simulink model "master_thesis_simulink"  (R2022a)
settings: Solver=VariableStepAuto  StartTime=0.0  StopTime=p_0p.time(end)  FixedStep=0.001  RelTol=1e-3
values from neighbouring files (symbols this model uses):
  markers_forearm = [0.00210510253906 -0.143263397217 -0.00798474121094]    [markers_forearm.mat]
  markers_shoulder = [0.010127746582 -0.151647644043 -0.0119686279297]    [markers_shoulder.mat]
undefined symbols (not defined in the file or in its folder): arm, DiscIntNeverNeededParam, Discrete, ekf, kf, LS, m, markers_hand, n, noise, q0, q0_LS, q0_model, sample_Time, selected, state_observer, Time, tSh_0_0Conf, X, Y, Z
libraries: sm_lib x2029, nesl_utility x1553, robotlib x75, ctrlSharedLib x8
(part 32 of 70)

== system master_thesis_simulink/Experiments/S2_F0_H2/Model validation/Human arm/Wrist_joint ==
  note: Experiments
  Constant : Constant  Value=0
  Constant1 : Constant  Value=0
  Constant2 : Constant  Value=0
  F_elbow__Wx : Subsystem
  PS-Simulink Converter{1..3,9..11} (6 alike) : nesl_utility/PS-Simulink Converter  PhysicalDomain=network_engine_domain  SubClassName=ps_output  LeftPortType=input  RightPortType=output  PseudoPeriodic=off  Frequencies=[]  VectorFormat=inherit  Unit=inherit  AffineConversion=off
      settings: SourceProductBaseCode=SS,PW,VE
  RighForeArm_rot1 : sm_lib/Frames and Transforms/Rigid Transform  TranslationMethod=Cartesian  TranslationStandardOffset=0  TranslationLengthUnit=m  TranslationStandardAxis=+Z  TranslationCartesianOffset=[0 0 -arm.forearm.radius+arm.hand.dimensions(3)/2]  TranslationROffset=0  TranslationROffsetUnits=m  TranslationZOffset=0  TranslationZOffsetUnits=m  TranslationThetaOffset=0  TranslationThetaOffsetUnits=deg  RotationMethod=None  RotationAngleUnits=rad  RotationStandardAxis=+Z  RotationAngle=pi/2  RotationArbitraryAxis=[1 0 0]  FollAlignAxisA=+X  BaseAlignAxisA=+Y  FollAlignAxisB=+Y  BaseAlignAxisB=+Z  RotationSequenceAxes=BaseAxes  RotationSequence=XYZ  RotationSequenceAngles=[pi/2, 0, 0]  RotationSequenceAnglesUnits=rad  RotationMatrix=[1 0 0; 0 1 0; 0 0 1]
  Wx_Wy : Subsystem
  Wy_Wz : Subsystem
  c1 : nesl_utility/Simulink-PS Converter  PhysicalDomain=network_engine_domain  SubClassName=ps_input  LeftPortType=input  RightPortType=output  PseudoPeriodic=off  Frequencies=[]  NoiseDistribution=none  NoiseParameters=[]  Unit=1  AffineConversion=off  FilteringAndDerivatives=filter  SimscapeFilterOrder=2  InputFilterTimeConstant=0.001  UdotUserProvided=0
      settings: SourceProductBaseCode=SS,PW,VE
  c2 : nesl_utility/Simulink-PS Converter  PhysicalDomain=network_engine_domain  SubClassName=ps_input  LeftPortType=input  RightPortType=output  PseudoPeriodic=off  Frequencies=[]  NoiseDistribution=none  NoiseParameters=[]  Unit=1  AffineConversion=off  FilteringAndDerivatives=filter  SimscapeFilterOrder=2  InputFilterTimeConstant=0.001  UdotUserProvided=0
      settings: SourceProductBaseCode=SS,PW,VE
  c3 : nesl_utility/Simulink-PS Converter  PhysicalDomain=network_engine_domain  SubClassName=ps_input  LeftPortType=input  RightPortType=output  PseudoPeriodic=off  Frequencies=[]  NoiseDistribution=none  NoiseParameters=[]  Unit=1  AffineConversion=off  FilteringAndDerivatives=filter  SimscapeFilterOrder=2  InputFilterTimeConstant=0.001  UdotUserProvided=0
      settings: SourceProductBaseCode=SS,PW,VE
  jRightWrist_rotx : sm_lib/Joints/Revolute Joint  JointMode=Normal  SenseConstraintForce=off  SenseConstraintForceX=off  SenseConstraintForceY=off  SenseConstraintForceZ=off  SenseConstraintTorque=off  SenseConstraintTorqueX=off  SenseConstraintTorqueY=off  SenseConstraintTorqueZ=off  SenseTotalForce=off  SenseTotalForceX=off  SenseTotalForceY=off  SenseTotalForceZ=off  SenseTotalTorque=off  SenseTotalTorqueX=off  SenseTotalTorqueY=off  SenseTotalTorqueZ=off  CompositeWrenchDir=FollowerOnBase  CompositeWrenchFrame=BaseFrame  EquilibriumPosition=0  EquilibriumPositionUnits=deg  SpringStiffness=0  SpringStiffnessUnits=N*m/deg  DampingCoefficient=0.01  DampingCoefficientUnits=kg*m^2/(rad*s)  TorqueActuationMode=ComputedTorque  MotionActuationMode=InputMotion  SensePosition=on  SenseVelocity=on  SenseAcceleration=off  SenseTorqueForce=off  SenseLowerLimitTorqueForce=off  SenseUpperLimitTorqueForce=off  LowerLimitSpecify=on  LowerLimitBound=-pi/4  LowerLimitBoundUnits=rad  LowerLimitStiffness=1e4  LowerLimitStiffnessUnits=N*m/deg  LowerLimitDamping=10  LowerLimitDampingUnits=N*m/(deg/s)  LowerLimitTransitionRegionWidth=0.1  LowerLimitTransitionRegionWidthUnits=deg  UpperLimitSpecify=on  UpperLimitBound=pi/3  UpperLimitBoundUnits=rad  UpperLimitStiffness=1e4  UpperLimitStiffnessUnits=N*m/deg  UpperLimitDamping=10  UpperLimitDampingUnits=N*m/(deg/s)  UpperLimitTransitionRegionWidth=0.1  UpperLimitTransitionRegionWidthUnits=deg  PositionTargetSpecify=on  PositionTargetPriority=High  PositionTargetValue=0  PositionTargetValueUnits=rad  VelocityTargetSpecify=off  VelocityTargetPriority=High  VelocityTargetValue=0  VelocityTargetValueUnits=deg/s
  jRightWrist_roty : sm_lib/Joints/Revolute Joint  JointMode=Normal  SenseConstraintForce=off  SenseConstraintForceX=off  SenseConstraintForceY=off  SenseConstraintForceZ=off  SenseConstraintTorque=off  SenseConstraintTorqueX=off  SenseConstraintTorqueY=off  SenseConstraintTorqueZ=off  SenseTotalForce=off  SenseTotalForceX=off  SenseTotalForceY=off  SenseTotalForceZ=off  SenseTotalTorque=off  SenseTotalTorqueX=off  SenseTotalTorqueY=off  SenseTotalTorqueZ=off  CompositeWrenchDir=FollowerOnBase  CompositeWrenchFrame=BaseFrame  EquilibriumPosition=0  EquilibriumPositionUnits=deg  SpringStiffness=0  SpringStiffnessUnits=N*m/deg  DampingCoefficient=0  DampingCoefficientUnits=kg*m^2/(rad*s)  TorqueActuationMode=ComputedTorque  MotionActuationMode=InputMotion  SensePosition=on  SenseVelocity=on  SenseAcceleration=off  SenseTorqueForce=off  SenseLowerLimitTorqueForce=off  SenseUpperLimitTorqueForce=off  LowerLimitSpecify=on  LowerLimitBound=-pi/10  LowerLimitBoundUnits=rad  LowerLimitStiffness=1e4  LowerLimitStiffnessUnits=N*m/deg  LowerLimitDamping=10  LowerLimitDampingUnits=N*m/(deg/s)  LowerLimitTransitionRegionWidth=0.1  LowerLimitTransitionRegionWidthUnits=deg  UpperLimitSpecify=on  UpperLimitBound=pi/10  UpperLimitBoundUnits=rad  UpperLimitStiffness=1e4  UpperLimitStiffnessUnits=N*m/deg  UpperLimitDamping=10  UpperLimitDampingUnits=N*m/(deg/s)  UpperLimitTransitionRegionWidth=0.1  UpperLimitTransitionRegionWidthUnits=deg  PositionTargetSpecify=on  PositionTargetPriority=High  PositionTargetValue=0  PositionTargetValueUnits=rad  VelocityTargetSpecify=off  VelocityTargetPriority=High  VelocityTargetValue=0  VelocityTargetValueUnits=deg/s
  jRightWrist_rotz : sm_lib/Joints/Revolute Joint  JointMode=Normal  SenseConstraintForce=off  SenseConstraintForceX=off  SenseConstraintForceY=off  SenseConstraintForceZ=off  SenseConstraintTorque=off  SenseConstraintTorqueX=off  SenseConstraintTorqueY=off  SenseConstraintTorqueZ=off  SenseTotalForce=off  SenseTotalForceX=off  SenseTotalForceY=off  SenseTotalForceZ=off  SenseTotalTorque=off  SenseTotalTorqueX=off  SenseTotalTorqueY=off  SenseTotalTorqueZ=off  CompositeWrenchDir=FollowerOnBase  CompositeWrenchFrame=BaseFrame  EquilibriumPosition=0  EquilibriumPositionUnits=deg  SpringStiffness=0  SpringStiffnessUnits=N*m/deg  DampingCoefficient=0  DampingCoefficientUnits=kg*m^2/(rad*s)  TorqueActuationMode=ComputedTorque  MotionActuationMode=InputMotion  SensePosition=on  SenseVelocity=on  SenseAcceleration=off  SenseTorqueForce=off  SenseLowerLimitTorqueForce=off  SenseUpperLimitTorqueForce=off  LowerLimitSpecify=on  LowerLimitBound=-20  LowerLimitBoundUnits=deg  LowerLimitStiffness=1e4  LowerLimitStiffnessUnits=N*m/deg  LowerLimitDamping=10  LowerLimitDampingUnits=N*m/(deg/s)  LowerLimitTransitionRegionWidth=0.1  LowerLimitTransitionRegionWidthUnits=deg  UpperLimitSpecify=on  UpperLimitBound=pi/6  UpperLimitBoundUnits=rad  UpperLimitStiffness=1e4  UpperLimitStiffnessUnits=N*m/deg  UpperLimitDamping=10  UpperLimitDampingUnits=N*m/(deg/s)  UpperLimitTransitionRegionWidth=0.1  UpperLimitTransitionRegionWidthUnits=deg  PositionTargetSpecify=on  PositionTargetPriority=High  PositionTargetValue=0  PositionTargetValueUnits=rad  VelocityTargetSpecify=off  VelocityTargetPriority=High  VelocityTargetValue=0  VelocityTargetValueUnits=deg/s
  B_wrist : PMIOPort  Side=Right
  F_elbow : PMIOPort  Port=2  Side=Left
  tag scope: q5=global, q6=global, q7=global, qdot5=global, qdot6=global, qdot7=global
  wires:
  Constant2/1 -> c3/1
  Constant1/1 -> c2/1
  Constant/1 -> c1/1
  PS-Simulink Converter3/1 -> [qdot7]
  PS-Simulink Converter2/1 -> [qdot6]
  PS-Simulink Converter1/1 -> [qdot5]
  PS-Simulink Converter9/1 -> [q5]
  PS-Simulink Converter10/1 -> [q6]
  PS-Simulink Converter11/1 -> [q7]
  connections:
  RighForeArm_rot1/LConn1 -- F_elbow/RConn1
  c3/RConn1 -- jRightWrist_rotz/LConn2
  c2/RConn1 -- jRightWrist_roty/LConn2
  c1/RConn1 -- jRightWrist_rotx/LConn2
  ?
  ?
  ?
  jRightWrist_rotz/RConn3 -- PS-Simulink Converter3/LConn1
  jRightWrist_roty/RConn3 -- PS-Simulink Converter2/LConn1
  jRightWrist_rotx/RConn3 -- PS-Simulink Converter1/LConn1
  B_wrist/RConn1 -- jRightWrist_rotz/RConn1
  F_elbow__Wx/LConn1 -- RighForeArm_rot1/RConn1
  jRightWrist_roty/RConn1 -- Wy_Wz/LConn1
  PS-Simulink Converter9/LConn1 -- jRightWrist_rotx/RConn2
  PS-Simulink Converter10/LConn1 -- jRightWrist_roty/RConn2
  jRightWrist_roty/LConn1 -- Wx_Wy/RConn1
  jRightWrist_rotz/RConn2 -- PS-Simulink Converter11/LConn1
  Wy_Wz/RConn1 -- jRightWrist_rotz/LConn1
  jRightWrist_rotx/RConn1 -- Wx_Wy/LConn1
  F_elbow__Wx/RConn1 -- jRightWrist_rotx/LConn1

== system master_thesis_simulink/Ros2Matlab/S0_F1_H2/Subscriber/M0/Odom ==
  Bus Selector : BusSelector  OutputSignals=Pose.Covariance
  Bus Selector1 : BusSelector  OutputSignals=Twist.Covariance
  Bus1 : BusSelector  OutputSignals=Twist.Twist.Linear.X,Twist.Twist.Linear.Y,Twist.Twist.Linear.Z
  Mux2 : Mux  Inputs=3
  Subscribe_odom : robotlib/Subscribe  topicSource=Select from ROS network  topic=/qualisys/Super_marker_0/odom  messageType=nav_msgs/Odometry  SampleTime=sample_Time  legacyBusStruct=off  messageQueueLength=1
  Terminator3 : Terminator
  v0_W : Outport
  Rp0_W : Outport  Port=2
  Rv0_W : Outport  Port=3
  wires:
  Bus1/3 -> Mux2/3  "<Z>"
  Bus1/1 -> Mux2/1  "<X>"
  Bus1/2 -> Mux2/2  "<Y>"
  Subscribe_odom/1 -> Terminator3/1
  Mux2/1 -> v0_W/1
  Subscribe_odom/2 -> Bus Selector1/1, Bus Selector/1, Bus1/1
  Bus Selector/1 -> Rp0_W/1  "<Covariance>"
  Bus Selector1/1 -> Rv0_W/1  "<Covariance>"

== system master_thesis_simulink/Ros2Matlab/S0_F1_H2/Subscriber/M0/Pose ==
  Bus Selector : BusSelector  OutputSignals=Pose.Orientation.W
  Bus Selector1 : BusSelector  OutputSignals=Pose.Orientation.X
  Bus Selector2 : BusSelector  OutputSignals=Pose.Orientation.Y
  Bus Selector3 : BusSelector  OutputSignals=Pose.Position.X,Pose.Position.Y,Pose.Position.Z
  Bus Selector4 : BusSelector  OutputSignals=Pose.Orientation.Z
  Mux1 : Mux  Inputs=3
  Mux2 : Mux
  Subscribe_pose : robotlib/Subscribe  topicSource=Select from ROS network  topic=/qualisys/Super_marker_0/pose  messageType=geometry_msgs/PoseStamped  SampleTime=sample_Time  legacyBusStruct=off  messageQueueLength=1
  quat_02W : Outport
  p0_W : Outport  Port=2
  tag scope: M0_isNew=global
  wires:
  Mux2/1 -> quat_02W/1
  Bus Selector4/1 -> Mux2/4  "<Z>"
  Mux1/1 -> p0_W/1
  Bus Selector3/3 -> Mux1/3  "<Z>"
  Bus Selector3/2 -> Mux1/2  "<Y>"
  Bus Selector3/1 -> Mux1/1  "<X>"
  Bus Selector2/1 -> Mux2/3  "<Y>"
  Bus Selector1/1 -> Mux2/2  "<X>"
  Bus Selector/1 -> Mux2/1  "<W>"
  Subscribe_pose/2 -> Bus Selector/1, Bus Selector1/1, Bus Selector2/1, Bus Selector3/1, Bus Selector4/1
  Subscribe_pose/1 -> [M0_isNew]

== system master_thesis_simulink/Ros2Matlab/S0_F1_H2/Subscriber/M2/Odom ==
  Bus1 : BusSelector  OutputSignals=Twist.Twist.Linear.X,Twist.Twist.Linear.Y,Twist.Twist.Linear.Z
  Bus2 : BusSelector  OutputSignals=Pose.Covariance
  Bus3 : BusSelector  OutputSignals=Twist.Covariance
  Mux2 : Mux  Inputs=3
  Subscribe_twist : robotlib/Subscribe  topicSource=Select from ROS network  topic=/qualisys/Super_marker_2/odom  messageType=nav_msgs/Odometry  SampleTime=sample_Time  legacyBusStruct=off  messageQueueLength=1
  Terminator3 : Terminator
  v2_W : Outport
  Rp2_W : Outport  Port=2
  Rv2_W : Outport  Port=3
  wires:
  Mux2/1 -> v2_W/1
  Subscribe_twist/1 -> Terminator3/1
  Bus1/2 -> Mux2/2  "<Y>"
  Bus1/1 -> Mux2/1  "<X>"
  Bus1/3 -> Mux2/3  "<Z>"
  Bus2/1 -> Rp2_W/1  "<Covariance>"
  Subscribe_twist/2 -> Bus3/1, Bus2/1, Bus1/1
  Bus3/1 -> Rv2_W/1  "<Covariance>"

== system master_thesis_simulink/Ros2Matlab/S0_F1_H2/Subscriber/M2/Pose ==
  Bus : BusSelector  OutputSignals=Pose.Position.X,Pose.Position.Y,Pose.Position.Z
  Mux : Mux  Inputs=3
  Subscribe_pose : robotlib/Subscribe  topicSource=Select from ROS network  topic=/qualisys/Super_marker_2/pose  messageType=geometry_msgs/PoseStamped  SampleTime=sample_Time  legacyBusStruct=off  messageQueueLength=1
  p2_W : Outport
  tag scope: M2_isNew=global
  wires:
  Bus/2 -> Mux/2  "<Y>"
  Bus/3 -> Mux/3  "<Z>"
  Subscribe_pose/2 -> Bus/1
  Mux/1 -> p2_W/1
  Bus/1 -> Mux/1  "<X>"
  Subscribe_pose/1 -> [M2_isNew]

== system master_thesis_simulink/Ros2Matlab/S0_F1_H2/Subscriber/M3/Odom ==
  Bus1 : BusSelector  OutputSignals=Twist.Twist.Linear.X,Twist.Twist.Linear.Y,Twist.Twist.Linear.Z
  Bus2 : BusSelector  OutputSignals=Pose.Covariance
  Bus3 : BusSelector  OutputSignals=Twist.Covariance
  Mux2 : Mux  Inputs=3
  Subscribe_twist : robotlib/Subscribe  topicSource=Select from ROS network  topic=/qualisys/Super_marker_3/odom  messageType=nav_msgs/Odometry  SampleTime=sample_Time  legacyBusStruct=off  messageQueueLength=1
  Terminator3 : Terminator
  v3_W : Outport
  Rp3_W : Outport  Port=2
  Rv3_W : Outport  Port=3
  wires:
  Bus1/3 -> Mux2/3  "<Z>"
  Bus1/1 -> Mux2/1  "<X>"
  Bus1/2 -> Mux2/2  "<Y>"
  Subscribe_twist/1 -> Terminator3/1
  Mux2/1 -> v3_W/1
  Bus2/1 -> Rp3_W/1  "<Covariance>"
  Subscribe_twist/2 -> Bus3/1, Bus2/1, Bus1/1
  Bus3/1 -> Rv3_W/1  "<Covariance>"

== system master_thesis_simulink/Ros2Matlab/S0_F1_H2/Subscriber/M3/Pose ==
  Bus : BusSelector  OutputSignals=Pose.Position.X,Pose.Position.Y,Pose.Position.Z
  Mux : Mux  Inputs=3
  Subscribe_pose : robotlib/Subscribe  topicSource=Select from ROS network  topic=/qualisys/Super_marker_3/pose  messageType=geometry_msgs/PoseStamped  SampleTime=sample_Time  legacyBusStruct=off  messageQueueLength=1
  p3_W : Outport
  tag scope: M3_isNew=global
  wires:
  Bus/1 -> Mux/1  "<X>"
  Mux/1 -> p3_W/1
  Subscribe_pose/2 -> Bus/1
  Bus/3 -> Mux/3  "<Z>"
  Bus/2 -> Mux/2  "<Y>"
  Subscribe_pose/1 -> [M3_isNew]

== system master_thesis_simulink/Ros2Matlab/S0_F1_H2/Subscriber/M4/Odom ==
  Bus1 : BusSelector  OutputSignals=Twist.Twist.Linear.X,Twist.Twist.Linear.Y,Twist.Twist.Linear.Z
  Bus2 : BusSelector  OutputSignals=Pose.Covariance
  Bus3 : BusSelector  OutputSignals=Twist.Covariance
  Mux2 : Mux  Inputs=3
  Subscribe_twist : robotlib/Subscribe  topicSource=Select from ROS network  topic=/qualisys/Super_marker_4/odom  messageType=nav_msgs/Odometry  SampleTime=sample_Time  legacyBusStruct=off  messageQueueLength=1
  Terminator3 : Terminator
  v4_W : Outport
  Rp4_W : Outport  Port=2
  Rv4_W : Outport  Port=3
  wires:
  Mux2/1 -> v4_W/1
  Subscribe_twist/1 -> Terminator3/1
  Bus1/2 -> Mux2/2  "<Y>"
  Bus1/1 -> Mux2/1  "<X>"
  Bus1/3 -> Mux2/3  "<Z>"
  Subscribe_twist/2 -> Bus3/1, Bus2/1, Bus1/1
  Bus2/1 -> Rp4_W/1  "<Covariance>"
  Bus3/1 -> Rv4_W/1  "<Covariance>"

== system master_thesis_simulink/Ros2Matlab/S0_F1_H2/Subscriber/M4/Pose ==
  Bus : BusSelector  OutputSignals=Pose.Position.X,Pose.Position.Y,Pose.Position.Z
  Mux : Mux  Inputs=3
  Subscribe_pose : robotlib/Subscribe  topicSource=Select from ROS network  topic=/qualisys/Super_marker_4/pose  messageType=geometry_msgs/PoseStamped  SampleTime=sample_Time  legacyBusStruct=off  messageQueueLength=1
  p4_W : Outport
  tag scope: M4_isNew=global
  wires:
  Bus/2 -> Mux/2  "<Y>"
  Bus/3 -> Mux/3  "<Z>"
  Subscribe_pose/2 -> Bus/1
  Mux/1 -> p4_W/1
  Bus/1 -> Mux/1  "<X>"
  Subscribe_pose/1 -> [M4_isNew]

== system master_thesis_simulink/Ros2Matlab/S0_F1_H2/Subscriber/Shoulder_RF/Pose ==
  Bus Selector : BusSelector  OutputSignals=Pose.Orientation.W
  Bus Selector1 : BusSelector  OutputSignals=Pose.Orientation.X
  Bus Selector2 : BusSelector  OutputSignals=Pose.Orientation.Y
  Bus Selector3 : BusSelector  OutputSignals=Pose.Position.X,Pose.Position.Y,Pose.Position.Z
  Bus Selector4 : BusSelector  OutputSignals=Pose.Orientation.Z
  Mux1 : Mux  Inputs=3
  Mux2 : Mux
  Subscribe_pose : robotlib/Subscribe  topicSource=Select from ROS network  topic=/qualisys/Shoulder_RF/pose  messageType=geometry_msgs/PoseStamped  SampleTime=sample_Time  legacyBusStruct=off  messageQueueLength=1
  quat_Sh2W : Outport
  pSh_W : Outport  Port=2
  tag scope: Sh_isNew=global
  wires:
  Mux2/1 -> quat_Sh2W/1
  Bus Selector4/1 -> Mux2/4  "<Z>"
  Mux1/1 -> pSh_W/1
  Bus Selector3/3 -> Mux1/3  "<Z>"
  Bus Selector3/2 -> Mux1/2  "<Y>"
  Bus Selector3/1 -> Mux1/1  "<X>"
  Bus Selector2/1 -> Mux2/3  "<Y>"
  Bus Selector1/1 -> Mux2/2  "<X>"
  Bus Selector/1 -> Mux2/1  "<W>"
  Subscribe_pose/2 -> Bus Selector/1, Bus Selector1/1, Bus Selector2/1, Bus Selector3/1, Bus Selector4/1
  Subscribe_pose/1 -> [Sh_isNew]

== system master_thesis_simulink/Ros2Matlab/S0_F2_H2/Subscriber/M0/Odom ==
  Bus Selector : BusSelector  OutputSignals=Pose.Covariance
  Bus Selector1 : BusSelector  OutputSignals=Twist.Covariance
  Bus1 : BusSelector  OutputSignals=Twist.Twist.Linear.X,Twist.Twist.Linear.Y,Twist.Twist.Linear.Z
  Mux2 : Mux  Inputs=3
  Subscribe_odom : robotlib/Subscribe  topicSource=Select from ROS network  topic=/qualisys/Super_marker_0/odom  messageType=nav_msgs/Odometry  SampleTime=sample_Time  legacyBusStruct=off  messageQueueLength=1
  Terminator3 : Terminator
  v0_W : Outport
  Rp0_W : Outport  Port=2
  Rv0_W : Outport  Port=3
  wires:
  Bus1/3 -> Mux2/3  "<Z>"
  Bus1/1 -> Mux2/1  "<X>"
  Bus1/2 -> Mux2/2  "<Y>"
  Subscribe_odom/1 -> Terminator3/1
  Mux2/1 -> v0_W/1
  Subscribe_odom/2 -> Bus Selector1/1, Bus Selector/1, Bus1/1
  Bus Selector/1 -> Rp0_W/1  "<Covariance>"
  Bus Selector1/1 -> Rv0_W/1  "<Covariance>"

== system master_thesis_simulink/Ros2Matlab/S0_F2_H2/Subscriber/M0/Pose ==
  Bus Selector : BusSelector  OutputSignals=Pose.Orientation.W
  Bus Selector1 : BusSelector  OutputSignals=Pose.Orientation.X
  Bus Selector2 : BusSelector  OutputSignals=Pose.Orientation.Y
  Bus Selector3 : BusSelector  OutputSignals=Pose.Position.X,Pose.Position.Y,Pose.Position.Z
  Bus Selector4 : BusSelector  OutputSignals=Pose.Orientation.Z
  Mux1 : Mux  Inputs=3
  Mux2 : Mux
  Subscribe_pose : robotlib/Subscribe  topicSource=Select from ROS network  topic=/qualisys/Super_marker_0/pose  messageType=geometry_msgs/PoseStamped  SampleTime=sample_Time  legacyBusStruct=off  messageQueueLength=1
  quat_02W : Outport
  p0_W : Outport  Port=2
  tag scope: M0_isNew=global
  wires:
  Mux2/1 -> quat_02W/1
  Bus Selector4/1 -> Mux2/4  "<Z>"
  Mux1/1 -> p0_W/1
  Bus Selector3/3 -> Mux1/3  "<Z>"
  Bus Selector3/2 -> Mux1/2  "<Y>"
  Bus Selector3/1 -> Mux1/1  "<X>"
  Bus Selector2/1 -> Mux2/3  "<Y>"
  Bus Selector1/1 -> Mux2/2  "<X>"
  Bus Selector/1 -> Mux2/1  "<W>"
  Subscribe_pose/2 -> Bus Selector/1, Bus Selector1/1, Bus Selector2/1, Bus Selector3/1, Bus Selector4/1
  Subscribe_pose/1 -> [M0_isNew]

== system master_thesis_simulink/Ros2Matlab/S0_F2_H2/Subscriber/M1/Odom ==
  Bus1 : BusSelector  OutputSignals=Twist.Twist.Linear.X,Twist.Twist.Linear.Y,Twist.Twist.Linear.Z
  Bus2 : BusSelector  OutputSignals=Pose.Covariance
  Bus3 : BusSelector  OutputSignals=Twist.Covariance
  Mux2 : Mux  Inputs=3
  Subscribe_twist : robotlib/Subscribe  topicSource=Select from ROS network  topic=/qualisys/Super_marker_1/odom  messageType=nav_msgs/Odometry  SampleTime=sample_Time  legacyBusStruct=off  messageQueueLength=1
  Terminator3 : Terminator
  v1_W : Outport
  Rp1_W : Outport  Port=2
  Rv1_W : Outport  Port=3
  wires:
  Bus1/3 -> Mux2/3  "<Z>"
  Bus1/1 -> Mux2/1  "<X>"
  Bus1/2 -> Mux2/2  "<Y>"
  Subscribe_twist/1 -> Terminator3/1
  Mux2/1 -> v1_W/1
  Subscribe_twist/2 -> Bus3/1, Bus2/1, Bus1/1
  Bus2/1 -> Rp1_W/1  "<Covariance>"
  Bus3/1 -> Rv1_W/1  "<Covariance>"

== system master_thesis_simulink/Ros2Matlab/S0_F2_H2/Subscriber/M1/Pose ==
  Bus : BusSelector  OutputSignals=Pose.Position.X,Pose.Position.Y,Pose.Position.Z
  Mux : Mux  Inputs=3
  Subscribe_pose : robotlib/Subscribe  topicSource=Select from ROS network  topic=/qualisys/Super_marker_1/pose  messageType=geometry_msgs/PoseStamped  SampleTime=sample_Time  legacyBusStruct=off  messageQueueLength=1
  p1_W : Outport
  tag scope: M1_isNew=global
  wires:
  Bus/1 -> Mux/1  "<X>"
  Mux/1 -> p1_W/1
  Subscribe_pose/2 -> Bus/1
  Bus/3 -> Mux/3  "<Z>"
  Bus/2 -> Mux/2  "<Y>"
  Subscribe_pose/1 -> [M1_isNew]

== system master_thesis_simulink/Ros2Matlab/S0_F2_H2/Subscriber/M2/Odom ==
  Bus1 : BusSelector  OutputSignals=Twist.Twist.Linear.X,Twist.Twist.Linear.Y,Twist.Twist.Linear.Z
  Bus2 : BusSelector  OutputSignals=Pose.Covariance
  Bus3 : BusSelector  OutputSignals=Twist.Covariance
  Mux2 : Mux  Inputs=3
  Subscribe_twist : robotlib/Subscribe  topicSource=Select from ROS network  topic=/qualisys/Super_marker_2/odom  messageType=nav_msgs/Odometry  SampleTime=sample_Time  legacyBusStruct=off  messageQueueLength=1
  Terminator3 : Terminator
  v2_W : Outport
  Rp2_W : Outport  Port=2
  Rv2_W : Outport  Port=3
  wires:
  Mux2/1 -> v2_W/1
  Subscribe_twist/1 -> Terminator3/1
  Bus1/2 -> Mux2/2  "<Y>"
  Bus1/1 -> Mux2/1  "<X>"
  Bus1/3 -> Mux2/3  "<Z>"
  Bus2/1 -> Rp2_W/1  "<Covariance>"
  Subscribe_twist/2 -> Bus3/1, Bus2/1, Bus1/1
  Bus3/1 -> Rv2_W/1  "<Covariance>"

== system master_thesis_simulink/Ros2Matlab/S0_F2_H2/Subscriber/M2/Pose ==
  Bus : BusSelector  OutputSignals=Pose.Position.X,Pose.Position.Y,Pose.Position.Z
  Mux : Mux  Inputs=3
  Subscribe_pose : robotlib/Subscribe  topicSource=Select from ROS network  topic=/qualisys/Super_marker_2/pose  messageType=geometry_msgs/PoseStamped  SampleTime=sample_Time  legacyBusStruct=off  messageQueueLength=1
  p2_W : Outport
  tag scope: M2_isNew=global
  wires:
  Bus/2 -> Mux/2  "<Y>"
  Bus/3 -> Mux/3  "<Z>"
  Subscribe_pose/2 -> Bus/1
  Mux/1 -> p2_W/1
  Bus/1 -> Mux/1  "<X>"
  Subscribe_pose/1 -> [M2_isNew]

== system master_thesis_simulink/Ros2Matlab/S0_F2_H2/Subscriber/M3/Odom ==
  Bus1 : BusSelector  OutputSignals=Twist.Twist.Linear.X,Twist.Twist.Linear.Y,Twist.Twist.Linear.Z
  Bus2 : BusSelector  OutputSignals=Pose.Covariance
  Bus3 : BusSelector  OutputSignals=Twist.Covariance
  Mux2 : Mux  Inputs=3
  Subscribe_twist : robotlib/Subscribe  topicSource=Select from ROS network  topic=/qualisys/Super_marker_3/odom  messageType=nav_msgs/Odometry  SampleTime=sample_Time  legacyBusStruct=off  messageQueueLength=1
  Terminator3 : Terminator
  v3_W : Outport
  Rp3_W : Outport  Port=2
  Rv3_W : Outport  Port=3
  wires:
  Bus1/3 -> Mux2/3  "<Z>"
  Bus1/1 -> Mux2/1  "<X>"
  Bus1/2 -> Mux2/2  "<Y>"
  Subscribe_twist/1 -> Terminator3/1
  Mux2/1 -> v3_W/1
  Bus2/1 -> Rp3_W/1  "<Covariance>"
  Subscribe_twist/2 -> Bus3/1, Bus2/1, Bus1/1
  Bus3/1 -> Rv3_W/1  "<Covariance>"

== system master_thesis_simulink/Ros2Matlab/S0_F2_H2/Subscriber/M3/Pose ==
  Bus : BusSelector  OutputSignals=Pose.Position.X,Pose.Position.Y,Pose.Position.Z
  Mux : Mux  Inputs=3
  Subscribe_pose : robotlib/Subscribe  topicSource=Select from ROS network  topic=/qualisys/Super_marker_3/pose  messageType=geometry_msgs/PoseStamped  SampleTime=sample_Time  legacyBusStruct=off  messageQueueLength=1
  p3_W : Outport
  tag scope: M3_isNew=global
  wires:
  Bus/1 -> Mux/1  "<X>"
  Mux/1 -> p3_W/1
  Subscribe_pose/2 -> Bus/1
  Bus/3 -> Mux/3  "<Z>"
  Bus/2 -> Mux/2  "<Y>"
  Subscribe_pose/1 -> [M3_isNew]

== system master_thesis_simulink/Ros2Matlab/S0_F2_H2/Subscriber/M4/Odom ==
  Bus1 : BusSelector  OutputSignals=Twist.Twist.Linear.X,Twist.Twist.Linear.Y,Twist.Twist.Linear.Z
  Bus2 : BusSelector  OutputSignals=Pose.Covariance
  Bus3 : BusSelector  OutputSignals=Twist.Covariance
  Mux2 : Mux  Inputs=3
  Subscribe_twist : robotlib/Subscribe  topicSource=Select from ROS network  topic=/qualisys/Super_marker_4/odom  messageType=nav_msgs/Odometry  SampleTime=sample_Time  legacyBusStruct=off  messageQueueLength=1
  Terminator3 : Terminator
  v4_W : Outport
  Rp4_W : Outport  Port=2
  Rv4_W : Outport  Port=3
  wires:
  Mux2/1 -> v4_W/1
  Subscribe_twist/1 -> Terminator3/1
  Bus1/2 -> Mux2/2  "<Y>"
  Bus1/1 -> Mux2/1  "<X>"
  Bus1/3 -> Mux2/3  "<Z>"
  Subscribe_twist/2 -> Bus3/1, Bus2/1, Bus1/1
  Bus2/1 -> Rp4_W/1  "<Covariance>"
  Bus3/1 -> Rv4_W/1  "<Covariance>"

== system master_thesis_simulink/Ros2Matlab/S0_F2_H2/Subscriber/M4/Pose ==
  Bus : BusSelector  OutputSignals=Pose.Position.X,Pose.Position.Y,Pose.Position.Z
  Mux : Mux  Inputs=3
  Subscribe_pose : robotlib/Subscribe  topicSource=Select from ROS network  topic=/qualisys/Super_marker_4/pose  messageType=geometry_msgs/PoseStamped  SampleTime=sample_Time  legacyBusStruct=off  messageQueueLength=1
  p4_W : Outport
  tag scope: M4_isNew=global
  wires:
  Bus/2 -> Mux/2  "<Y>"
  Bus/3 -> Mux/3  "<Z>"
  Subscribe_pose/2 -> Bus/1
  Mux/1 -> p4_W/1
  Bus/1 -> Mux/1  "<X>"
  Subscribe_pose/1 -> [M4_isNew]

== system master_thesis_simulink/Ros2Matlab/S0_F2_H2/Subscriber/Shoulder_RF/Pose ==
  Bus Selector : BusSelector  OutputSignals=Pose.Orientation.W
  Bus Selector1 : BusSelector  OutputSignals=Pose.Orientation.X
  Bus Selector2 : BusSelector  OutputSignals=Pose.Orientation.Y
  Bus Selector3 : BusSelector  OutputSignals=Pose.Position.X,Pose.Position.Y,Pose.Position.Z
  Bus Selector4 : BusSelector  OutputSignals=Pose.Orientation.Z
  Mux1 : Mux  Inputs=3
  Mux2 : Mux
  Subscribe_pose : robotlib/Subscribe  topicSource=Select from ROS network  topic=/qualisys/Shoulder_RF/pose  messageType=geometry_msgs/PoseStamped  SampleTime=sample_Time  legacyBusStruct=off  messageQueueLength=1
  quat_Sh2W : Outport
  pSh_W : Outport  Port=2
  tag scope: Sh_isNew=global
  wires:
  Mux2/1 -> quat_Sh2W/1
  Bus Selector4/1 -> Mux2/4  "<Z>"
  Mux1/1 -> pSh_W/1
  Bus Selector3/3 -> Mux1/3  "<Z>"
  Bus Selector3/2 -> Mux1/2  "<Y>"
  Bus Selector3/1 -> Mux1/1  "<X>"
  Bus Selector2/1 -> Mux2/3  "<Y>"
  Bus Selector1/1 -> Mux2/2  "<X>"
  Bus Selector/1 -> Mux2/1  "<W>"
  Subscribe_pose/2 -> Bus Selector/1, Bus Selector1/1, Bus Selector2/1, Bus Selector3/1, Bus Selector4/1
  Subscribe_pose/1 -> [Sh_isNew]

== system master_thesis_simulink/Ros2Matlab/S1_F0_H2/Subscriber/M0/Odom ==
  Bus Selector : BusSelector  OutputSignals=Pose.Covariance
  Bus Selector1 : BusSelector  OutputSignals=Twist.Covariance
  Bus1 : BusSelector  OutputSignals=Twist.Twist.Linear.X,Twist.Twist.Linear.Y,Twist.Twist.Linear.Z
  Mux2 : Mux  Inputs=3
  Subscribe_odom : robotlib/Subscribe  topicSource=Select from ROS network  topic=/qualisys/Super_marker_0/odom  messageType=nav_msgs/Odometry  SampleTime=sample_Time  legacyBusStruct=off  messageQueueLength=1
  Terminator3 : Terminator
  v0_W : Outport
  Rp0_W : Outport  Port=2
  Rv0_W : Outport  Port=3
  wires:
  Bus1/3 -> Mux2/3  "<Z>"
  Bus1/1 -> Mux2/1  "<X>"
  Bus1/2 -> Mux2/2  "<Y>"
  Subscribe_odom/1 -> Terminator3/1
  Mux2/1 -> v0_W/1
  Subscribe_odom/2 -> Bus Selector1/1, Bus Selector/1, Bus1/1
  Bus Selector/1 -> Rp0_W/1  "<Covariance>"
  Bus Selector1/1 -> Rv0_W/1  "<Covariance>"

== system master_thesis_simulink/Ros2Matlab/S1_F0_H2/Subscriber/M0/Pose ==
  Bus Selector : BusSelector  OutputSignals=Pose.Orientation.W
  Bus Selector1 : BusSelector  OutputSignals=Pose.Orientation.X
  Bus Selector2 : BusSelector  OutputSignals=Pose.Orientation.Y
  Bus Selector3 : BusSelector  OutputSignals=Pose.Position.X,Pose.Position.Y,Pose.Position.Z
  Bus Selector4 : BusSelector  OutputSignals=Pose.Orientation.Z
  Mux1 : Mux  Inputs=3
  Mux2 : Mux
  Subscribe_pose : robotlib/Subscribe  topicSource=Select from ROS network  topic=/qualisys/Super_marker_0/pose  messageType=geometry_msgs/PoseStamped  SampleTime=sample_Time  legacyBusStruct=off  messageQueueLength=1
  quat_02W : Outport
  p0_W : Outport  Port=2
  tag scope: M0_isNew=global
  wires:
  Mux2/1 -> quat_02W/1
  Bus Selector4/1 -> Mux2/4  "<Z>"
  Mux1/1 -> p0_W/1
  Bus Selector3/3 -> Mux1/3  "<Z>"
  Bus Selector3/2 -> Mux1/2  "<Y>"
  Bus Selector3/1 -> Mux1/1  "<X>"
  Bus Selector2/1 -> Mux2/3  "<Y>"
  Bus Selector1/1 -> Mux2/2  "<X>"
  Bus Selector/1 -> Mux2/1  "<W>"
  Subscribe_pose/2 -> Bus Selector/1, Bus Selector1/1, Bus Selector2/1, Bus Selector3/1, Bus Selector4/1
  Subscribe_pose/1 -> [M0_isNew]

== system master_thesis_simulink/Ros2Matlab/S1_F0_H2/Subscriber/M1/Odom ==
  Bus1 : BusSelector  OutputSignals=Twist.Twist.Linear.X,Twist.Twist.Linear.Y,Twist.Twist.Linear.Z
  Bus2 : BusSelector  OutputSignals=Pose.Covariance
  Bus3 : BusSelector  OutputSignals=Twist.Covariance
  Mux2 : Mux  Inputs=3
  Subscribe_twist : robotlib/Subscribe  topicSource=Select from ROS network  topic=/qualisys/Super_marker_1/odom  messageType=nav_msgs/Odometry  SampleTime=sample_Time  legacyBusStruct=off  messageQueueLength=1
  Terminator3 : Terminator
  v1_W : Outport
  Rp1_W : Outport  Port=2
  Rv1_W : Outport  Port=3
  wires:
  Bus1/3 -> Mux2/3  "<Z>"
  Bus1/1 -> Mux2/1  "<X>"
  Bus1/2 -> Mux2/2  "<Y>"
  Subscribe_twist/1 -> Terminator3/1
  Mux2/1 -> v1_W/1
  Subscribe_twist/2 -> Bus3/1, Bus2/1, Bus1/1
  Bus2/1 -> Rp1_W/1  "<Covariance>"
  Bus3/1 -> Rv1_W/1  "<Covariance>"

== system master_thesis_simulink/Ros2Matlab/S1_F0_H2/Subscriber/M1/Pose ==
  Bus : BusSelector  OutputSignals=Pose.Position.X,Pose.Position.Y,Pose.Position.Z
  Mux : Mux  Inputs=3
  Subscribe_pose : robotlib/Subscribe  topicSource=Select from ROS network  topic=/qualisys/Super_marker_1/pose  messageType=geometry_msgs/PoseStamped  SampleTime=sample_Time  legacyBusStruct=off  messageQueueLength=1
  p1_W : Outport
  tag scope: M1_isNew=global
  wires:
  Bus/1 -> Mux/1  "<X>"
  Mux/1 -> p1_W/1
  Subscribe_pose/2 -> Bus/1
  Bus/3 -> Mux/3  "<Z>"
  Bus/2 -> Mux/2  "<Y>"
  Subscribe_pose/1 -> [M1_isNew]

== system master_thesis_simulink/Ros2Matlab/S1_F0_H2/Subscriber/M3/Odom ==
  Bus1 : BusSelector  OutputSignals=Twist.Twist.Linear.X,Twist.Twist.Linear.Y,Twist.Twist.Linear.Z
  Bus2 : BusSelector  OutputSignals=Pose.Covariance
  Bus3 : BusSelector  OutputSignals=Twist.Covariance
  Mux2 : Mux  Inputs=3
  Subscribe_twist : robotlib/Subscribe  topicSource=Select from ROS network  topic=/qualisys/Super_marker_3/odom  messageType=nav_msgs/Odometry  SampleTime=sample_Time  legacyBusStruct=off  messageQueueLength=1
  Terminator3 : Terminator
  v3_W : Outport
  Rp3_W : Outport  Port=2
  Rv3_W : Outport  Port=3
  wires:
  Bus1/3 -> Mux2/3  "<Z>"
  Bus1/1 -> Mux2/1  "<X>"
  Bus1/2 -> Mux2/2  "<Y>"
  Subscribe_twist/1 -> Terminator3/1
  Mux2/1 -> v3_W/1
  Bus2/1 -> Rp3_W/1  "<Covariance>"
  Subscribe_twist/2 -> Bus3/1, Bus2/1, Bus1/1
  Bus3/1 -> Rv3_W/1  "<Covariance>"

== system master_thesis_simulink/Ros2Matlab/S1_F0_H2/Subscriber/M3/Pose ==
  Bus : BusSelector  OutputSignals=Pose.Position.X,Pose.Position.Y,Pose.Position.Z
  Mux : Mux  Inputs=3
  Subscribe_pose : robotlib/Subscribe  topicSource=Select from ROS network  topic=/qualisys/Super_marker_3/pose  messageType=geometry_msgs/PoseStamped  SampleTime=sample_Time  legacyBusStruct=off  messageQueueLength=1
  p3_W : Outport
  tag scope: M3_isNew=global
  wires:
  Bus/1 -> Mux/1  "<X>"
  Mux/1 -> p3_W/1
  Subscribe_pose/2 -> Bus/1
  Bus/3 -> Mux/3  "<Z>"
  Bus/2 -> Mux/2  "<Y>"
  Subscribe_pose/1 -> [M3_isNew]

== system master_thesis_simulink/Ros2Matlab/S1_F0_H2/Subscriber/M4/Odom ==
  Bus1 : BusSelector  OutputSignals=Twist.Twist.Linear.X,Twist.Twist.Linear.Y,Twist.Twist.Linear.Z
  Bus2 : BusSelector  OutputSignals=Pose.Covariance
  Bus3 : BusSelector  OutputSignals=Twist.Covariance
  Mux2 : Mux  Inputs=3
  Subscribe_twist : robotlib/Subscribe  topicSource=Select from ROS network  topic=/qualisys/Super_marker_4/odom  messageType=nav_msgs/Odometry  SampleTime=sample_Time  legacyBusStruct=off  messageQueueLength=1
  Terminator3 : Terminator
  v4_W : Outport
  Rp4_W : Outport  Port=2
  Rv4_W : Outport  Port=3
  wires:
  Mux2/1 -> v4_W/1
  Subscribe_twist/1 -> Terminator3/1
  Bus1/2 -> Mux2/2  "<Y>"
  Bus1/1 -> Mux2/1  "<X>"
  Bus1/3 -> Mux2/3  "<Z>"
  Subscribe_twist/2 -> Bus3/1, Bus2/1, Bus1/1
  Bus2/1 -> Rp4_W/1  "<Covariance>"
  Bus3/1 -> Rv4_W/1  "<Covariance>"

== system master_thesis_simulink/Ros2Matlab/S1_F0_H2/Subscriber/M4/Pose ==
  Bus : BusSelector  OutputSignals=Pose.Position.X,Pose.Position.Y,Pose.Position.Z
  Mux : Mux  Inputs=3
  Subscribe_pose : robotlib/Subscribe  topicSource=Select from ROS network  topic=/qualisys/Super_marker_4/pose  messageType=geometry_msgs/PoseStamped  SampleTime=sample_Time  legacyBusStruct=off  messageQueueLength=1
  p4_W : Outport
  tag scope: M4_isNew=global
  wires:
  Bus/2 -> Mux/2  "<Y>"
  Bus/3 -> Mux/3  "<Z>"
  Subscribe_pose/2 -> Bus/1
  Mux/1 -> p4_W/1
  Bus/1 -> Mux/1  "<X>"
  Subscribe_pose/1 -> [M4_isNew]

== system master_thesis_simulink/Ros2Matlab/S1_F0_H2/Subscriber/Shoulder_RF/Pose ==
  Bus Selector : BusSelector  OutputSignals=Pose.Orientation.W
  Bus Selector1 : BusSelector  OutputSignals=Pose.Orientation.X
  Bus Selector2 : BusSelector  OutputSignals=Pose.Orientation.Y
  Bus Selector3 : BusSelector  OutputSignals=Pose.Position.X,Pose.Position.Y,Pose.Position.Z
  Bus Selector4 : BusSelector  OutputSignals=Pose.Orientation.Z
  Mux1 : Mux  Inputs=3
  Mux2 : Mux
  Subscribe_pose : robotlib/Subscribe  topicSource=Select from ROS network  topic=/qualisys/Shoulder_RF/pose  messageType=geometry_msgs/PoseStamped  SampleTime=sample_Time  legacyBusStruct=off  messageQueueLength=1
  quat_Sh2W : Outport
  pSh_W : Outport  Port=2
  tag scope: Sh_isNew=global
  wires:
  Mux2/1 -> quat_Sh2W/1
  Bus Selector4/1 -> Mux2/4  "<Z>"
  Mux1/1 -> pSh_W/1
  Bus Selector3/3 -> Mux1/3  "<Z>"
  Bus Selector3/2 -> Mux1/2  "<Y>"
  Bus Selector3/1 -> Mux1/1  "<X>"
  Bus Selector2/1 -> Mux2/3  "<Y>"
  Bus Selector1/1 -> Mux2/2  "<X>"
  Bus Selector/1 -> Mux2/1  "<W>"
  Subscribe_pose/2 -> Bus Selector/1, Bus Selector1/1, Bus Selector2/1, Bus Selector3/1, Bus Selector4/1
  Subscribe_pose/1 -> [Sh_isNew]

== system master_thesis_simulink/Ros2Matlab/S1_F0_H3/Subscriber/M0/Odom ==
  Bus Selector : BusSelector  OutputSignals=Pose.Covariance
  Bus Selector1 : BusSelector  OutputSignals=Twist.Covariance
  Bus1 : BusSelector  OutputSignals=Twist.Twist.Linear.X,Twist.Twist.Linear.Y,Twist.Twist.Linear.Z
  Mux2 : Mux  Inputs=3
  Subscribe_odom : robotlib/Subscribe  topicSource=Select from ROS network  topic=/qualisys/Super_marker_0/odom  messageType=nav_msgs/Odometry  SampleTime=sample_Time  legacyBusStruct=off  messageQueueLength=1
  Terminator3 : Terminator
  v0_W : Outport
  Rp0_W : Outport  Port=2
  Rv0_W : Outport  Port=3
  wires:
  Bus1/3 -> Mux2/3  "<Z>"
  Bus1/1 -> Mux2/1  "<X>"
  Bus1/2 -> Mux2/2  "<Y>"
  Subscribe_odom/1 -> Terminator3/1
  Mux2/1 -> v0_W/1
  Subscribe_odom/2 -> Bus Selector1/1, Bus Selector/1, Bus1/1
  Bus Selector/1 -> Rp0_W/1  "<Covariance>"
  Bus Selector1/1 -> Rv0_W/1  "<Covariance>"

== system master_thesis_simulink/Ros2Matlab/S1_F0_H3/Subscriber/M0/Pose ==
  Bus Selector : BusSelector  OutputSignals=Pose.Orientation.W
  Bus Selector1 : BusSelector  OutputSignals=Pose.Orientation.X
  Bus Selector2 : BusSelector  OutputSignals=Pose.Orientation.Y
  Bus Selector3 : BusSelector  OutputSignals=Pose.Position.X,Pose.Position.Y,Pose.Position.Z
  Bus Selector4 : BusSelector  OutputSignals=Pose.Orientation.Z
  Mux1 : Mux  Inputs=3
  Mux2 : Mux
  Subscribe_pose : robotlib/Subscribe  topicSource=Select from ROS network  topic=/qualisys/Super_marker_0/pose  messageType=geometry_msgs/PoseStamped  SampleTime=sample_Time  legacyBusStruct=off  messageQueueLength=1
  quat_02W : Outport
  p0_W : Outport  Port=2
  tag scope: M0_isNew=global
  wires:
  Mux2/1 -> quat_02W/1
  Bus Selector4/1 -> Mux2/4  "<Z>"
  Mux1/1 -> p0_W/1
  Bus Selector3/3 -> Mux1/3  "<Z>"
  Bus Selector3/2 -> Mux1/2  "<Y>"
  Bus Selector3/1 -> Mux1/1  "<X>"
  Bus Selector2/1 -> Mux2/3  "<Y>"
  Bus Selector1/1 -> Mux2/2  "<X>"
  Bus Selector/1 -> Mux2/1  "<W>"
  Subscribe_pose/2 -> Bus Selector/1, Bus Selector1/1, Bus Selector2/1, Bus Selector3/1, Bus Selector4/1
  Subscribe_pose/1 -> [M0_isNew]

== system master_thesis_simulink/Ros2Matlab/S1_F0_H3/Subscriber/M1/Odom ==
  Bus1 : BusSelector  OutputSignals=Twist.Twist.Linear.X,Twist.Twist.Linear.Y,Twist.Twist.Linear.Z
  Bus2 : BusSelector  OutputSignals=Pose.Covariance
  Bus3 : BusSelector  OutputSignals=Twist.Covariance
  Mux2 : Mux  Inputs=3
  Subscribe_twist : robotlib/Subscribe  topicSource=Select from ROS network  topic=/qualisys/Super_marker_1/odom  messageType=nav_msgs/Odometry  SampleTime=sample_Time  legacyBusStruct=off  messageQueueLength=1
  Terminator3 : Terminator
  v1_W : Outport
  Rp1_W : Outport  Port=2
  Rv1_W : Outport  Port=3
  wires:
  Bus1/3 -> Mux2/3  "<Z>"
  Bus1/1 -> Mux2/1  "<X>"
  Bus1/2 -> Mux2/2  "<Y>"
  Subscribe_twist/1 -> Terminator3/1
  Mux2/1 -> v1_W/1
  Subscribe_twist/2 -> Bus3/1, Bus2/1, Bus1/1
  Bus2/1 -> Rp1_W/1  "<Covariance>"
  Bus3/1 -> Rv1_W/1  "<Covariance>"

== system master_thesis_simulink/Ros2Matlab/S1_F0_H3/Subscriber/M1/Pose ==
  Bus : BusSelector  OutputSignals=Pose.Position.X,Pose.Position.Y,Pose.Position.Z
  Mux : Mux  Inputs=3
  Subscribe_pose : robotlib/Subscribe  topicSource=Select from ROS network  topic=/qualisys/Super_marker_1/pose  messageType=geometry_msgs/PoseStamped  SampleTime=sample_Time  legacyBusStruct=off  messageQueueLength=1
  p1_W : Outport
  tag scope: M1_isNew=global
  wires:
  Bus/1 -> Mux/1  "<X>"
  Mux/1 -> p1_W/1
  Subscribe_pose/2 -> Bus/1
  Bus/3 -> Mux/3  "<Z>"
  Bus/2 -> Mux/2  "<Y>"
  Subscribe_pose/1 -> [M1_isNew]

== system master_thesis_simulink/Ros2Matlab/S1_F0_H3/Subscriber/M2/Odom ==
  Bus1 : BusSelector  OutputSignals=Twist.Twist.Linear.X,Twist.Twist.Linear.Y,Twist.Twist.Linear.Z
  Bus2 : BusSelector  OutputSignals=Pose.Covariance
  Bus3 : BusSelector  OutputSignals=Twist.Covariance
  Mux2 : Mux  Inputs=3
  Subscribe_twist : robotlib/Subscribe  topicSource=Select from ROS network  topic=/qualisys/Super_marker_2/odom  messageType=nav_msgs/Odometry  SampleTime=sample_Time  legacyBusStruct=off  messageQueueLength=1
  Terminator3 : Terminator
  v2_W : Outport
  Rp2_W : Outport  Port=2
  Rv2_W : Outport  Port=3
  wires:
  Mux2/1 -> v2_W/1
  Subscribe_twist/1 -> Terminator3/1
  Bus1/2 -> Mux2/2  "<Y>"
  Bus1/1 -> Mux2/1  "<X>"
  Bus1/3 -> Mux2/3  "<Z>"
  Bus2/1 -> Rp2_W/1  "<Covariance>"
  Subscribe_twist/2 -> Bus3/1, Bus2/1, Bus1/1
  Bus3/1 -> Rv2_W/1  "<Covariance>"

== system master_thesis_simulink/Ros2Matlab/S1_F0_H3/Subscriber/M2/Pose ==
  Bus : BusSelector  OutputSignals=Pose.Position.X,Pose.Position.Y,Pose.Position.Z
  Mux : Mux  Inputs=3
  Subscribe_pose : robotlib/Subscribe  topicSource=Select from ROS network  topic=/qualisys/Super_marker_2/pose  messageType=geometry_msgs/PoseStamped  SampleTime=sample_Time  legacyBusStruct=off  messageQueueLength=1
  p2_W : Outport
  tag scope: M2_isNew=global
  wires:
  Bus/2 -> Mux/2  "<Y>"
  Bus/3 -> Mux/3  "<Z>"
  Subscribe_pose/2 -> Bus/1
  Mux/1 -> p2_W/1
  Bus/1 -> Mux/1  "<X>"
  Subscribe_pose/1 -> [M2_isNew]

== system master_thesis_simulink/Ros2Matlab/S1_F0_H3/Subscriber/M3/Odom ==
  Bus1 : BusSelector  OutputSignals=Twist.Twist.Linear.X,Twist.Twist.Linear.Y,Twist.Twist.Linear.Z
  Bus2 : BusSelector  OutputSignals=Pose.Covariance
  Bus3 : BusSelector  OutputSignals=Twist.Covariance
  Mux2 : Mux  Inputs=3
  Subscribe_twist : robotlib/Subscribe  topicSource=Select from ROS network  topic=/qualisys/Super_marker_3/odom  messageType=nav_msgs/Odometry  SampleTime=sample_Time  legacyBusStruct=off  messageQueueLength=1
  Terminator3 : Terminator
  v3_W : Outport
  Rp3_W : Outport  Port=2
  Rv3_W : Outport  Port=3
  wires:
  Bus1/3 -> Mux2/3  "<Z>"
  Bus1/1 -> Mux2/1  "<X>"
  Bus1/2 -> Mux2/2  "<Y>"
  Subscribe_twist/1 -> Terminator3/1
  Mux2/1 -> v3_W/1
  Bus2/1 -> Rp3_W/1  "<Covariance>"
  Subscribe_twist/2 -> Bus3/1, Bus2/1, Bus1/1
  Bus3/1 -> Rv3_W/1  "<Covariance>"

== system master_thesis_simulink/Ros2Matlab/S1_F0_H3/Subscriber/M3/Pose ==
  Bus : BusSelector  OutputSignals=Pose.Position.X,Pose.Position.Y,Pose.Position.Z
  Mux : Mux  Inputs=3
  Subscribe_pose : robotlib/Subscribe  topicSource=Select from ROS network  topic=/qualisys/Super_marker_3/pose  messageType=geometry_msgs/PoseStamped  SampleTime=sample_Time  legacyBusStruct=off  messageQueueLength=1
  p3_W : Outport
  tag scope: M3_isNew=global
  wires:
  Bus/1 -> Mux/1  "<X>"
  Mux/1 -> p3_W/1
  Subscribe_pose/2 -> Bus/1
  Bus/3 -> Mux/3  "<Z>"
  Bus/2 -> Mux/2  "<Y>"
  Subscribe_pose/1 -> [M3_isNew]

== system master_thesis_simulink/Ros2Matlab/S1_F0_H3/Subscriber/M4/Odom ==
  Bus1 : BusSelector  OutputSignals=Twist.Twist.Linear.X,Twist.Twist.Linear.Y,Twist.Twist.Linear.Z
  Bus2 : BusSelector  OutputSignals=Pose.Covariance
  Bus3 : BusSelector  OutputSignals=Twist.Covariance
  Mux2 : Mux  Inputs=3
  Subscribe_twist : robotlib/Subscribe  topicSource=Select from ROS network  topic=/qualisys/Super_marker_4/odom  messageType=nav_msgs/Odometry  SampleTime=sample_Time  legacyBusStruct=off  messageQueueLength=1
  Terminator3 : Terminator
  v4_W : Outport
  Rp4_W : Outport  Port=2
  Rv4_W : Outport  Port=3
  wires:
  Mux2/1 -> v4_W/1
  Subscribe_twist/1 -> Terminator3/1
  Bus1/2 -> Mux2/2  "<Y>"
  Bus1/1 -> Mux2/1  "<X>"
  Bus1/3 -> Mux2/3  "<Z>"
  Subscribe_twist/2 -> Bus3/1, Bus2/1, Bus1/1
  Bus2/1 -> Rp4_W/1  "<Covariance>"
  Bus3/1 -> Rv4_W/1  "<Covariance>"

== system master_thesis_simulink/Ros2Matlab/S1_F0_H3/Subscriber/M4/Pose ==
  Bus : BusSelector  OutputSignals=Pose.Position.X,Pose.Position.Y,Pose.Position.Z
  Mux : Mux  Inputs=3
  Subscribe_pose : robotlib/Subscribe  topicSource=Select from ROS network  topic=/qualisys/Super_marker_4/pose  messageType=geometry_msgs/PoseStamped  SampleTime=sample_Time  legacyBusStruct=off  messageQueueLength=1
  p4_W : Outport
  tag scope: M4_isNew=global
  wires:
  Bus/2 -> Mux/2  "<Y>"
  Bus/3 -> Mux/3  "<Z>"
  Subscribe_pose/2 -> Bus/1
  Mux/1 -> p4_W/1
  Bus/1 -> Mux/1  "<X>"
  Subscribe_pose/1 -> [M4_isNew]

== system master_thesis_simulink/Ros2Matlab/S1_F0_H3/Subscriber/Shoulder_RF/Pose ==
  Bus Selector : BusSelector  OutputSignals=Pose.Orientation.W
  Bus Selector1 : BusSelector  OutputSignals=Pose.Orientation.X
  Bus Selector2 : BusSelector  OutputSignals=Pose.Orientation.Y
  Bus Selector3 : BusSelector  OutputSignals=Pose.Position.X,Pose.Position.Y,Pose.Position.Z
  Bus Selector4 : BusSelector  OutputSignals=Pose.Orientation.Z
  Mux1 : Mux  Inputs=3
  Mux2 : Mux
  Subscribe_pose : robotlib/Subscribe  topicSource=Select from ROS network  topic=/qualisys/Shoulder_RF/pose  messageType=geometry_msgs/PoseStamped  SampleTime=sample_Time  legacyBusStruct=off  messageQueueLength=1
  quat_Sh2W : Outport
  pSh_W : Outport  Port=2
  tag scope: Sh_isNew=global
  wires:
  Mux2/1 -> quat_Sh2W/1
  Bus Selector4/1 -> Mux2/4  "<Z>"
  Mux1/1 -> pSh_W/1
  Bus Selector3/3 -> Mux1/3  "<Z>"
  Bus Selector3/2 -> Mux1/2  "<Y>"
  Bus Selector3/1 -> Mux1/1  "<X>"
  Bus Selector2/1 -> Mux2/3  "<Y>"
  Bus Selector1/1 -> Mux2/2  "<X>"
  Bus Selector/1 -> Mux2/1  "<W>"
  Subscribe_pose/2 -> Bus Selector/1, Bus Selector1/1, Bus Selector2/1, Bus Selector3/1, Bus Selector4/1
  Subscribe_pose/1 -> [Sh_isNew]

== system master_thesis_simulink/Ros2Matlab/S1_F1_H2/Subscriber/M0/Odom ==
  Bus Selector : BusSelector  OutputSignals=Pose.Covariance
  Bus Selector1 : BusSelector  OutputSignals=Twist.Covariance
  Bus1 : BusSelector  OutputSignals=Twist.Twist.Linear.X,Twist.Twist.Linear.Y,Twist.Twist.Linear.Z
  Mux2 : Mux  Inputs=3
  Subscribe_odom : robotlib/Subscribe  topicSource=Select from ROS network  topic=/qualisys/Super_marker_0/odom  messageType=nav_msgs/Odometry  SampleTime=sample_Time  legacyBusStruct=off  messageQueueLength=1
  Terminator3 : Terminator
  v0_W : Outport
  Rp0_W : Outport  Port=2
  Rv0_W : Outport  Port=3
  wires:
  Bus1/3 -> Mux2/3  "<Z>"
  Bus1/1 -> Mux2/1  "<X>"
  Bus1/2 -> Mux2/2  "<Y>"
  Subscribe_odom/1 -> Terminator3/1
  Mux2/1 -> v0_W/1
  Subscribe_odom/2 -> Bus Selector1/1, Bus Selector/1, Bus1/1
  Bus Selector/1 -> Rp0_W/1  "<Covariance>"
  Bus Selector1/1 -> Rv0_W/1  "<Covariance>"

== system master_thesis_simulink/Ros2Matlab/S1_F1_H2/Subscriber/M0/Pose ==
  Bus Selector : BusSelector  OutputSignals=Pose.Orientation.W
  Bus Selector1 : BusSelector  OutputSignals=Pose.Orientation.X
  Bus Selector2 : BusSelector  OutputSignals=Pose.Orientation.Y
  Bus Selector3 : BusSelector  OutputSignals=Pose.Position.X,Pose.Position.Y,Pose.Position.Z
  Bus Selector4 : BusSelector  OutputSignals=Pose.Orientation.Z
  Mux1 : Mux  Inputs=3
  Mux2 : Mux
  Subscribe_pose : robotlib/Subscribe  topicSource=Select from ROS network  topic=/qualisys/Super_marker_0/pose  messageType=geometry_msgs/PoseStamped  SampleTime=sample_Time  legacyBusStruct=off  messageQueueLength=1
  quat_02W : Outport
  p0_W : Outport  Port=2
  tag scope: M0_isNew=global
  wires:
  Mux2/1 -> quat_02W/1
  Bus Selector4/1 -> Mux2/4  "<Z>"
  Mux1/1 -> p0_W/1
  Bus Selector3/3 -> Mux1/3  "<Z>"
  Bus Selector3/2 -> Mux1/2  "<Y>"
  Bus Selector3/1 -> Mux1/1  "<X>"
  Bus Selector2/1 -> Mux2/3  "<Y>"
  Bus Selector1/1 -> Mux2/2  "<X>"
  Bus Selector/1 -> Mux2/1  "<W>"
  Subscribe_pose/2 -> Bus Selector/1, Bus Selector1/1, Bus Selector2/1, Bus Selector3/1, Bus Selector4/1
  Subscribe_pose/1 -> [M0_isNew]

== system master_thesis_simulink/Ros2Matlab/S1_F1_H2/Subscriber/M1/Odom ==
  Bus1 : BusSelector  OutputSignals=Twist.Twist.Linear.X,Twist.Twist.Linear.Y,Twist.Twist.Linear.Z
  Bus2 : BusSelector  OutputSignals=Pose.Covariance
  Bus3 : BusSelector  OutputSignals=Twist.Covariance
  Mux2 : Mux  Inputs=3
  Subscribe_twist : robotlib/Subscribe  topicSource=Select from ROS network  topic=/qualisys/Super_marker_1/odom  messageType=nav_msgs/Odometry  SampleTime=sample_Time  legacyBusStruct=off  messageQueueLength=1
  Terminator3 : Terminator
  v1_W : Outport
  Rp1_W : Outport  Port=2
  Rv1_W : Outport  Port=3
  wires:
  Bus1/3 -> Mux2/3  "<Z>"
  Bus1/1 -> Mux2/1  "<X>"
  Bus1/2 -> Mux2/2  "<Y>"
  Subscribe_twist/1 -> Terminator3/1
  Mux2/1 -> v1_W/1
  Subscribe_twist/2 -> Bus3/1, Bus2/1, Bus1/1
  Bus2/1 -> Rp1_W/1  "<Covariance>"
  Bus3/1 -> Rv1_W/1  "<Covariance>"

== system master_thesis_simulink/Ros2Matlab/S1_F1_H2/Subscriber/M1/Pose ==
  Bus : BusSelector  OutputSignals=Pose.Position.X,Pose.Position.Y,Pose.Position.Z
  Mux : Mux  Inputs=3
  Subscribe_pose : robotlib/Subscribe  topicSource=Select from ROS network  topic=/qualisys/Super_marker_1/pose  messageType=geometry_msgs/PoseStamped  SampleTime=sample_Time  legacyBusStruct=off  messageQueueLength=1
  p1_W : Outport
  tag scope: M1_isNew=global
  wires:
  Bus/1 -> Mux/1  "<X>"
  Mux/1 -> p1_W/1
  Subscribe_pose/2 -> Bus/1
  Bus/3 -> Mux/3  "<Z>"
  Bus/2 -> Mux/2  "<Y>"
  Subscribe_pose/1 -> [M1_isNew]

== system master_thesis_simulink/Ros2Matlab/S1_F1_H2/Subscriber/M2/Odom ==
  Bus1 : BusSelector  OutputSignals=Twist.Twist.Linear.X,Twist.Twist.Linear.Y,Twist.Twist.Linear.Z
  Bus2 : BusSelector  OutputSignals=Pose.Covariance
  Bus3 : BusSelector  OutputSignals=Twist.Covariance
  Mux2 : Mux  Inputs=3
  Subscribe_twist : robotlib/Subscribe  topicSource=Select from ROS network  topic=/qualisys/Super_marker_2/odom  messageType=nav_msgs/Odometry  SampleTime=sample_Time  legacyBusStruct=off  messageQueueLength=1
  Terminator3 : Terminator
  v2_W : Outport
  Rp2_W : Outport  Port=2
  Rv2_W : Outport  Port=3
  wires:
  Mux2/1 -> v2_W/1
  Subscribe_twist/1 -> Terminator3/1
  Bus1/2 -> Mux2/2  "<Y>"
  Bus1/1 -> Mux2/1  "<X>"
  Bus1/3 -> Mux2/3  "<Z>"
  Bus2/1 -> Rp2_W/1  "<Covariance>"
  Subscribe_twist/2 -> Bus3/1, Bus2/1, Bus1/1
  Bus3/1 -> Rv2_W/1  "<Covariance>"

== system master_thesis_simulink/Ros2Matlab/S1_F1_H2/Subscriber/M2/Pose ==
  Bus : BusSelector  OutputSignals=Pose.Position.X,Pose.Position.Y,Pose.Position.Z
  Mux : Mux  Inputs=3
  Subscribe_pose : robotlib/Subscribe  topicSource=Select from ROS network  topic=/qualisys/Super_marker_2/pose  messageType=geometry_msgs/PoseStamped  SampleTime=sample_Time  legacyBusStruct=off  messageQueueLength=1
  p2_W : Outport
  tag scope: M2_isNew=global
  wires:
  Bus/2 -> Mux/2  "<Y>"
  Bus/3 -> Mux/3  "<Z>"
  Subscribe_pose/2 -> Bus/1
  Mux/1 -> p2_W/1
  Bus/1 -> Mux/1  "<X>"
  Subscribe_pose/1 -> [M2_isNew]

== system master_thesis_simulink/Ros2Matlab/S1_F1_H2/Subscriber/M3/Odom ==
  Bus1 : BusSelector  OutputSignals=Twist.Twist.Linear.X,Twist.Twist.Linear.Y,Twist.Twist.Linear.Z
  Bus2 : BusSelector  OutputSignals=Pose.Covariance
  Bus3 : BusSelector  OutputSignals=Twist.Covariance
  Mux2 : Mux  Inputs=3
  Subscribe_twist : robotlib/Subscribe  topicSource=Select from ROS network  topic=/qualisys/Super_marker_3/odom  messageType=nav_msgs/Odometry  SampleTime=sample_Time  legacyBusStruct=off  messageQueueLength=1
  Terminator3 : Terminator
  v3_W : Outport
  Rp3_W : Outport  Port=2
  Rv3_W : Outport  Port=3
  wires:
  Bus1/3 -> Mux2/3  "<Z>"
  Bus1/1 -> Mux2/1  "<X>"
  Bus1/2 -> Mux2/2  "<Y>"
  Subscribe_twist/1 -> Terminator3/1
  Mux2/1 -> v3_W/1
  Bus2/1 -> Rp3_W/1  "<Covariance>"
  Subscribe_twist/2 -> Bus3/1, Bus2/1, Bus1/1
  Bus3/1 -> Rv3_W/1  "<Covariance>"
